simulink model "test"  (R2024a)
settings: Solver=VariableStepAuto  StartTime=0.0  StopTime=10.0  FixedStep=0.0001  RelTol=8e-4
libraries: simulink x6
settings Model: Creator=18311  LastModifiedBy=18311

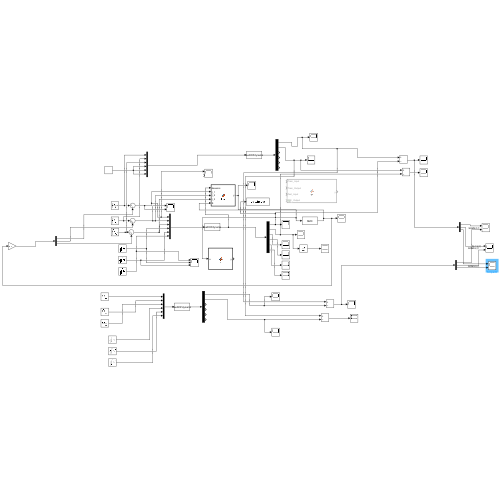
[thumbnail: Simulink's stored preview of the top-level diagram]
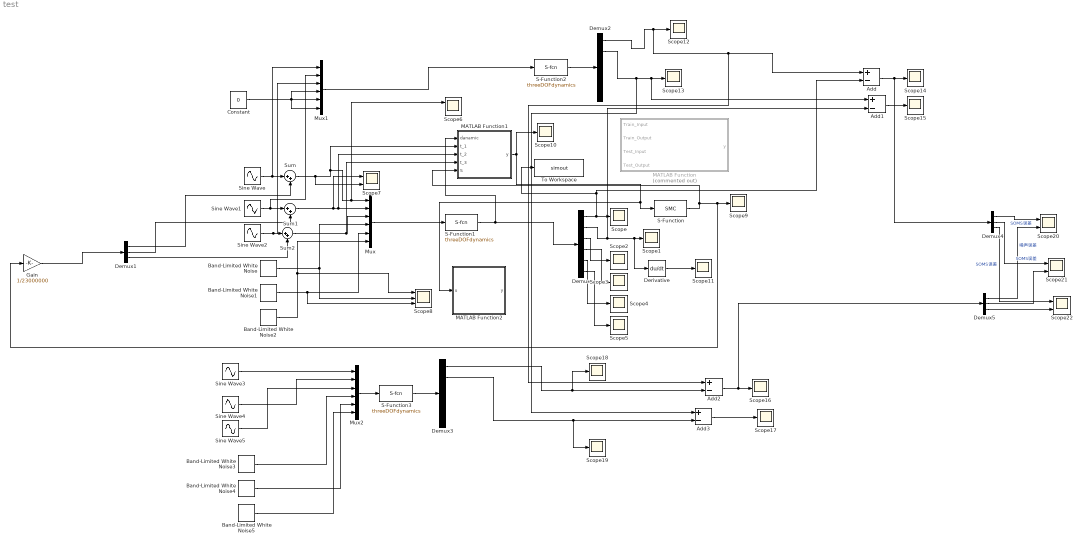
== system test ==
  Add{,1..3} (4 alike) : Sum  Inputs=+-
  Band-Limited White Noise : simulink/Sources/Band-Limited White Noise  Cov=[0.00000000005]  Ts=0.01  seed=[23341]
  Band-Limited White Noise1 : simulink/Sources/Band-Limited White Noise  Cov=[0.00000000005]  Ts=0.01  seed=[12345]
  Band-Limited White Noise2 : simulink/Sources/Band-Limited White Noise  Cov=[0.00000000005]  Ts=0.01  seed=[4356]
  Band-Limited White Noise3 : simulink/Sources/Band-Limited White Noise  Cov=[0.00000000005]  Ts=0.01  seed=[23341]
  Band-Limited White Noise4 : simulink/Sources/Band-Limited White Noise  Cov=[0.00000000005]  Ts=0.01  seed=[12345]
  Band-Limited White Noise5 : simulink/Sources/Band-Limited White Noise  Cov=[0.00000000005]  Ts=0.01  seed=[4356]
  Constant : Constant  Value=0
  Demux : Demux  Outputs=6
  Demux1 : Demux  Outputs=3
  Demux2 : Demux  Outputs=6
  Demux3 : Demux  Outputs=6
  Demux4 : Demux  Outputs=3
  Demux5 : Demux  Outputs=3
  Derivative : Derivative
  Gain : Gain  Gain=1/23000000
  MATLAB Function : MATLAB Function  Commented=on  TreatAsAtomicUnit=on
  MATLAB Function1 : MATLAB Function  TreatAsAtomicUnit=on
  MATLAB Function2 : MATLAB Function  TreatAsAtomicUnit=on
  Mux : Mux  Inputs=6
  Mux1 : Mux  Inputs=6
  Mux2 : Mux  Inputs=6
  S-Function : S-Function  FunctionName=SMC  SFunctionDeploymentMode=off  EnableBusSupport=off
  S-Function1 : S-Function  FunctionName=threeDOFdynamics  SFunctionDeploymentMode=off  EnableBusSupport=off
  S-Function2 : S-Function  FunctionName=threeDOFdynamics  SFunctionDeploymentMode=off  EnableBusSupport=off
  S-Function3 : S-Function  FunctionName=threeDOFdynamics  SFunctionDeploymentMode=off  EnableBusSupport=off
  Scope{,1..5,9..19} (17 alike) : Scope
  Scope{6..7,20..22} (5 alike) : Scope  NumInputPorts=2
  Scope8 : Scope  NumInputPorts=3
  Sine Wave : Sin  Amplitude=0.0003  Bias=0.0003  Phase=-pi/2  SampleTime=0
  Sine Wave{1..2,4..5} (4 alike) : Sin  Amplitude=0.01  Bias=0.01  Phase=-pi/2  SampleTime=0
  Sine Wave3 : Sin  Amplitude=0.0003  Bias=0.0003  Phase=-pi/2  SampleTime=0
  Sum : Sum  Inputs=|++
  Sum1 : Sum  Inputs=|++
  Sum2 : Sum  Inputs=|++
  To Workspace : ToWorkspace  VariableName=simout  SampleTime=-1
  wires:
  Sum/1 -> Scope7/2, MATLAB Function1/2(t_1), Scope6/1, Mux/1
  Sum1/1 -> Scope7/1, MATLAB Function1/3(t_2), Mux/2
  Sum2/1 -> MATLAB Function1/4(t_3), Mux/3
  Mux/1 -> S-Function1/1
  S-Function1/1 -> MATLAB Function1/1(danamic), Demux/1
  Demux/1 -> Add/2, To Workspace/1, Scope/1
  Demux/2 -> Derivative/1, Scope1/1, Add1/2
  Demux/3 -> Scope2/1
  Demux/4 -> Scope3/1
  Demux/5 -> Scope4/1
  Demux/6 -> Scope5/1
  MATLAB Function1/1(y) -> Scope10/1, MATLAB Function2/1(u), S-Function/1
  S-Function/1 -> Gain/1, Scope9/1, MATLAB Function1/5(S)
  Derivative/1 -> Scope11/1
  Sine Wave/1 -> Mux1/1, Sum/1
  Sine Wave1/1 -> Mux1/2, Sum1/1
  Sine Wave2/1 -> Mux1/3, Sum2/1
  Band-Limited White Noise/1 -> Mux/4, Scope8/2
  Band-Limited White Noise2/1 -> Mux/6, Scope8/1
  Gain/1 -> Demux1/1
  Band-Limited White Noise1/1 -> Scope8/3, Mux/5
  Demux1/1 -> Sum/2
  Demux1/2 -> Sum1/2
  Demux1/3 -> Sum2/2
  Constant/1 -> Mux1/4, Mux1/6, Mux1/5
  Mux1/1 -> S-Function2/1
  S-Function2/1 -> Demux2/1
  Demux2/1 -> Add2/1, Add/1, Scope12/1
  Demux2/2 -> Add3/1, Add1/1, Scope13/1
  Mux2/1 -> S-Function3/1
  Sine Wave3/1 -> Mux2/1
  Sine Wave4/1 -> Mux2/2
  Sine Wave5/1 -> Mux2/3
  Band-Limited White Noise3/1 -> Mux2/4
  Band-Limited White Noise4/1 -> Mux2/5
  Band-Limited White Noise5/1 -> Mux2/6
  S-Function3/1 -> Demux3/1
  Demux3/1 -> Add2/2, Scope18/1
  Demux3/2 -> Scope19/1, Add3/2
  Add/1 -> Demux4/1, Scope14/1
  Add1/1 -> Scope15/1
  Add2/1 -> Demux5/1, Scope16/1
  Add3/1 -> Scope17/1
  Demux4/1 -> Scope20/1  "SOMS误差"
  Demux5/1 -> Scope20/2  "噪声误差"
  Demux4/2 -> Scope21/1  "SOMS误差"
  Demux5/2 -> Scope21/2
  Demux4/3 -> Scope22/1  "SOMS误差"
  Demux5/3 -> Scope22/2

== matlab function test/MATLAB Function1 ==
  data: danamic input; y output; t_1 input; t_2 input; t_3 input; S input
function y = fcn(danamic, t_1, t_2, t_3, S)

y = zeros(12,1);
y(1) = danamic(1);
y(2) = danamic(2);
y(3) = t_1;
y(4) = danamic(4);
y(5) = danamic(5);
y(6) = t_2;
y(7) = danamic(7);
y(8) = danamic(8);
y(9) = t_3;
y(10) = S(1);
y(11) = S(2);
y(12) = S(3);

== matlab function test/MATLAB Function ==
  data: Train_Input input; y output; Train_Output input; Test_Input input; Test_Output input
function y = fcn(Train_Input, Train_Output, Test_Input, Test_Output)
% suppose the Input is [q1, q1_dot, torque1, q2, q2_dot, torque2, q3, q3_dot, torque3]
% suppose the Output is [q1, q1_dot, torque1, q2, q2_dot, torque2, q3, q3_dot, torque3]

% M is inertia Matrix
M = [1, 1, 1;
     1, 1, 1;
     1, 1, 1];
A = [-10, 0, -10;
     0,  -10, 0;
     0,   0, -10];

Train_Loop = size(Train_Input, 2);
Test_Loop  = size(Test_Input,  2);

%initial the friction matrix F and load disturbance matrix tau
F_Train    = zeros(3, Train_Loop);
F_Test     = zeros(3, Test_Loop);
tua_Train  = zeros(3, Train_Loop); 
tua_Test   = zeros(3, Test_Loop);
phi_1_Train= zeros(3, Train_Loop);
phi_1_Test = zeros(3, Train_Loop);
phi_2_Train= zeros(3, Train_Loop);
phi_2_Test = zeros(3, Train_Loop);

x_tilde_1_Train = zeros(3, Train_Loop);
x_tilde_2_Train = zeros(3, Train_Loop);
x_tilde_3_Train = zeros(3, Train_Loop);
% x_tilde_1_Test  = zeros(3, Test_Loop);
% x_tilde_2_Test  = zeros(3, Test_Loop);
% x_tilde_3_Test  = zeros(3, Test_Loop);

%inpur x overline
x_overline_1_Train = zeros(3, Train_Loop);
x_overline_2_Train = zeros(3, Train_Loop);
x_overline_3_Train = zeros(3, Train_Loop);
%output x overline
x_overline_1_Test  = zeros(3, Train_Loop);
x_overline_2_Test  = zeros(3, Train_Loop);
x_overline_3_Test  = zeros(3, Train_Loop);



for i = 1:1:Train_Loop
    F_Train(:,i) = [1.1*Train_Input(i, 2) + 0.3*sin(3*Train_Input(i, 1));
                    1.2*Train_Input(i, 5) + 0.4*sin(3*Train_Input(i, 4));
                    1.4*Train_Input(i, 8) + 0.3*sin(3*Train_Input(i, 7))];
    tua_Train(:,i) = [0.2  * sin(Train_Input(i, 2));
                      0.1  * sin(Train_Input(i, 5));
                      0.15 * sin(Train_Input(i, 8))];
    x_overline_1_Train(:,i) = [Train_Input(i, 1);
                               Train_Input(i, 2);
                               Train_Input(i, 3)];
    x_overline_2_Train(:,i) = [Train_Input(i, 4);
                               Train_Input(i, 5);
                               Train_Input(i, 6)];
    x_overline_3_Train(:,i) = [Train_Input(i, 7);
                               Train_Input(i, 8);
                               Train_Input(i, 9)];
    phi_1_Train(:,i) = [10*Train_Input(i, 1)^3     + 0.5*Train_Input(i, 5)  + 10*Train_Input(i, 7);
                        1.24*Train_Input(i, 4)     + 0.04*Train_Input(i, 5) + 0.6*sin(Train_Input(i, 8))
                        0.6*sin(Train_Input(i, 1)) + 5*Train_Input(i, 7)    + 3*sin(Train_Input(i, 7))];
    phi_2_Train(:,i) = [50*Train_Input(i, 1)^3     + 0.5*Train_Input(i, 5)  + 20*Train_Input(i, 7);
                        7.44*Train_Input(i, 4)     + 0.24*Train_Input(i, 5) + 3.6*sin(Train_Input(i, 8))
                        56*sin(Train_Input(i, 1))  + 70*Train_Input(i, 7)^2 + 1.05*sin(Train_Input(i, 7))];
end

for i = 1:1:Test_Loop
    F_Test(:,i) = [1.1*Test_Input(i, 2) + 0.3*sin(3*Test_Input(i, 1));
                   1.2*Test_Input(i, 5) + 0.4*sin(3*Test_Input(i, 4));
                   1.4*Test_Input(i, 8) + 0.3*sin(3*Test_Input(i, 7))];
    tua_Test(:,i) = [0.2  * sin(Test_Input(i, 2));
                     0.1  * sin(Test_Input(i, 5));
                     0.15 * sin(Test_Input(i, 8))];
    x_overline_1_Test(:,i) = [Test_Output(i, 1);
                              Test_Output(i, 2);
                              Test_Output(i, 3)];
    x_overline_2_Test(:,i) = [Test_Output(i, 4);
                              Test_Output(i, 5);
                              Test_Output(i, 6)];
    x_overline_3_Test(:,i) = [Test_Output(i, 7);
                              Test_Output(i, 8);
                              Test_Output(i, 9)];
    phi_1_Test(:,i) = [10*Test_Input(i, 1)^3     + 0.5*Test_Input(i, 5)  + 10*Test_Input(i, 7);
                       1.24*Test_Input(i, 4)     + 0.04*Test_Input(i, 5) + 0.6*sin(Test_Input(i, 8))
                       0.6*sin(Test_Input(i, 1)) + 5*Test_Input(i, 7)    + 3*sin(Test_Input(i, 7))];
    phi_2_Test(:,i) = [50*Test_Input(i, 1)^3     + 0.5*Test_Input(i, 5)  + 20*Test_Input(i, 7);
                       7.44*Test_Input(i, 4)     + 0.24*Test_Input(i, 5) + 3.6*sin(Test_Input(i, 8))
                       56*sin(Test_Input(i, 1))  + 70*Test_Input(i, 7)^2 + 1.05*sin(Test_Input(i, 7))];
end

mu_Train = M * (- F_Train - tau_Train);
% mu_Test  = M * (- F_Test - tua_Test);

% Initial neural network strucure
Input_Layer  = 3;
Hidden_Layer = 4;
Output_Layer = 3;

% Layer_Output_1 = zeros(Hidden_Layer, 1);
% Layer_Output_2 = zeros(Hidden_Layer, 1);
% Layer_Output_3 = zeros(Hidden_Layer, 1);

% Initial neural network weights
W_hat_1 = ones(Output_Layer, Hidden_Layer);
V_hat_1 = ones(Hidden_Layer, Input_Layer);
W_hat_2 = ones(Output_Layer, Hidden_Layer);
V_hat_2 = ones(Hidden_Layer, Input_Layer);
W_hat_3 = ones(Output_Layer, Hidden_Layer);
V_hat_3 = ones(Hidden_Layer, Input_Layer);


% Train neural network
for L = 1:1:Train_Loop
    Layer_Output_1_Train = W_hat_1 * sigmoidM(V_hat_1 * x_overline_1_Train);
    Layer_Output_2_Train = W_hat_2 * sigmoidM(V_hat_2 * x_overline_2_Train);
    Layer_Output_3_Train = W_hat_3 * sigmoidM(V_hat_3 * x_overline_3_Train);

    x_tilde_1_Train  = A * x_tilde_1_Train + mu_Train + phi_1_Train - Layer_Output_1_Train + x_tilde_1_Train; 
    x_tilde_2_Train  = A * x_tilde_2_Train + mu_Train + phi_1_Train - Layer_Output_2_Train + x_tilde_2_Train; 
    x_tilde_3_Train  = A * x_tilde_3_Train + mu_Train + phi_1_Train - Layer_Output_3_Train + x_tilde_3_Train; 
    
    W_hat_1 = W_hat_1 - alpha_1 * (x_tilde_1_Train.' * A^(-1)).' * (sigmoidM(V_hat_1 * x_overline_1_Train)).' - rho_1*norm(x_tilde_1_Train)*W_hat_1;
    V_hat_1 = V_hat_1 - alpha_2 * (x_tilde_1_Train.' * A^(-1) * W_hat_1 * (I - diag(sigmoidM(V_hat_1*x_tilde_1_Train)^2))).' * x_overline_1_Train.' - rho_2 * norm(x_tilde_1_Train)*V_hat_1;
end

% Neural network test
for L = 1:1:Test_Loop
    Layer_Output_1_Test = W_hat_1 * sigmoidM(V_hat_1 * x_overline_1_Train);
    Layer_Output_2_Test = W_hat_2 * sigmoidM(V_hat_2 * x_overline_2_Train);
    Layer_Output_3_Test = W_hat_3 * sigmoidM(V_hat_3 * x_overline_3_Train);    
end

differnece_1 = (Layer_Output_1_Test - x_overline_1_Test)/x_overline_1_Test
differnece_2 = (Layer_Output_2_Test - x_overline_2_Test)/x_overline_2_Test
differnece_3 = (Layer_Output_3_Test - x_overline_3_Test)/x_overline_3_Test

end



function y = sigmoid(x)
    y = 1/(1+exp(-x));
end


function y = sigmoidM(x)
    y = zeros(size(x,1), size(x,2));
    for i = 1:1:size(x,1)
        for ii = 1:1:size(x,2)
            y(i,ii) = sigmoid(x(i, ii));
        end
    end
end

== matlab function test/MATLAB Function2 ==
  data: u input; y output
function y = fcn(u)

y = zeros(3, 1);

y   = [10*u(1)^3+0.5*u(5)+10*u(7);
       1.24*u(4)+0.04*u(5)+0.6*sin(u(8));
       0.6*sin(u(1))+5*u(7)+3*sin(u(7))];
